simulink model "Converter_With_Parasitics_efficiency"  (R2024a)
settings: Solver=VariableStepAuto  StartTime=0.0  StopTime=0.2  RelTol=1e-3
libraries: spsSeriesRLCBranchLib x3, spsCurrentMeasurementLib x2, spsVoltageMeasurementLib x2, spsDiodeLib x1, spsMosfetLib x1, sps_lib x1, spsDCVoltageSourceLib x1
settings Model: Creator=DELL  LastModifiedBy=DELL

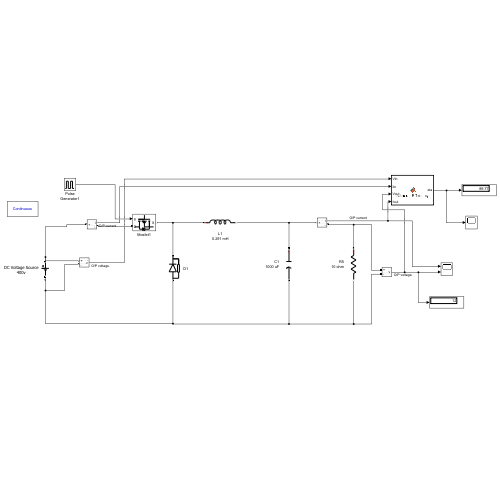
[thumbnail: Simulink's stored preview of the top-level diagram]
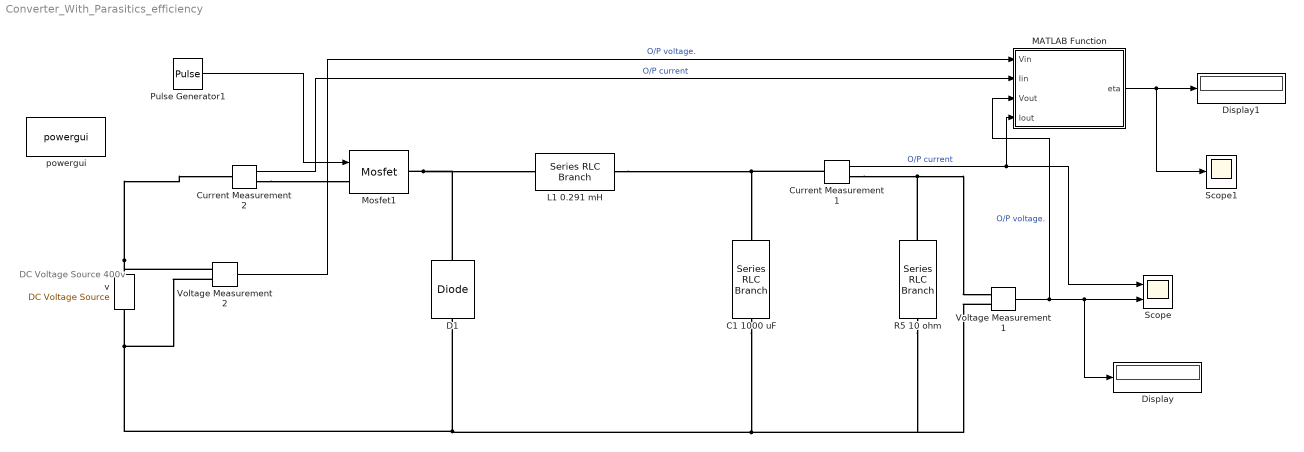
== system Converter_With_Parasitics_efficiency ==
  note: DC Voltage Source
      | 400v
  C1 1000 uF : spsSeriesRLCBranchLib/Series RLC Branch  LConnTagsString=__new0  RConnTagsString=__new0  BranchType=C  Resistance=1  Inductance=1e-3  SetiL0=off  InitialCurrent=0  Capacitance=100e-6  Setx0=off  InitialVoltage=0  Measurements=None
  Current Measurement1 : spsCurrentMeasurementLib/Current Measurement  PhasorSimulation=off  OutputType=Complex  PSBequivalent=0
  Current Measurement2 : spsCurrentMeasurementLib/Current Measurement  PhasorSimulation=off  OutputType=Complex  PSBequivalent=0
  D1 : spsDiodeLib/Diode  Ron=0.001  Lon=0  Vf=0.8  IC=0  UseSnubber=0  Rs=500  Cs=250e-9  Measurements=off
  Display : Display
  Display1 : Display
  L1 0.291 mH : spsSeriesRLCBranchLib/Series RLC Branch  LConnTagsString=__new0  RConnTagsString=__new0  BranchType=L  Resistance=1  Inductance=0.291e-3  SetiL0=off  InitialCurrent=0  Capacitance=1e-6  Setx0=off  InitialVoltage=0  Measurements=None
  MATLAB Function : MATLAB Function  TreatAsAtomicUnit=on
  Mosfet1 : spsMosfetLib/Mosfet  Ron=0.1  Lon=0  Rd=0.01  Vfd=0  IC=0  Rs=1e5  Cs=inf  Measurements=off
  Pulse Generator1 : DiscretePulseGenerator  PulseType=Time based  Period=1/200000  PulseWidth=3.1947
  R5 10 ohm : spsSeriesRLCBranchLib/Series RLC Branch  LConnTagsString=__new0  RConnTagsString=__new0  BranchType=R  Resistance=10  Inductance=1e-3  SetiL0=off  InitialCurrent=0  Capacitance=100e-6  Setx0=off  InitialVoltage=0  Measurements=None
  Scope : Scope  NumInputPorts=2
  Scope1 : Scope
  Voltage Measurement1 : spsVoltageMeasurementLib/Voltage Measurement  PhasorSimulation=off  OutputType=Complex  PSBequivalent=0
  Voltage Measurement2 : spsVoltageMeasurementLib/Voltage Measurement  PhasorSimulation=off  OutputType=Complex  PSBequivalent=0
  powergui : sps_lib/powergui  Priority=1  SimulationMode=Continuous  SampleTime=50e-6  frequency=60  Iterations=50  frequencyindice=0  Pbase=100e6  ErrMax=1e-4  UnitsV=kV  UnitsW=MW  buscounter=0  FunctionMessages=off  echomessages=off  EnableUseOfTLC=off  CurrentSourceSwitches=off  DisableSnubberDevices=off  DisableRonSwitches=off  DisableVfSwitches=off  DisplayEquations=off  AutomaticDiscreteSolvers=off  SolverType=Tustin/Backward Euler (TBE)  Interpol=off  ExternalGateDelay=off  methode=off  Ts=100  x0status=blocks  SPID=on  SwTol=0  HookPort=off  NonlinearTolerance=1e-4  nMaxIteration=100  ContinueOnMaxIteration=off  RestoreLinks=warning  ResistiveCurrentMeasurement=off  Frange=[0:2:500]  Ylog=off  Xlog=on  ShowGrid=off  save=off  variable=ZData  structure=0  ZoomFFT=off  StartTime=0.0  cycles=1  DisplayStyle=1  fundamental=60  FreqAxis=off  MaxFrequency=1000  frequencyindicesteady=1  RmsSteady=1  display=off
  v : spsDCVoltageSourceLib/DC Voltage Source  Amplitude=400  Measurements=None
  wires:
  Pulse Generator1/1 -> Mosfet1/1
  Current Measurement1/1 -> MATLAB Function/4(Iout), Scope/1  "O/P current"
  Voltage Measurement1/1 -> MATLAB Function/3(Vout), Display/1, Scope/2  "O/P voltage."
  Current Measurement2/1 -> MATLAB Function/2(Iin)  "O/P current"
  Voltage Measurement2/1 -> MATLAB Function/1(Vin)  "O/P voltage."
  MATLAB Function/1(eta) -> Scope1/1, Display1/1
  connections:
  L1 0.291 mH/RConn1 -- Current Measurement1/LConn1 -- C1 1000 uF/LConn1
  C1 1000 uF/RConn1 -- D1/LConn1 -- v/LConn1 -- Voltage Measurement2/LConn2 -- Voltage Measurement1/LConn2 -- R5 10 ohm/RConn1
  Mosfet1/RConn1 -- L1 0.291 mH/LConn1 -- D1/RConn1
  Current Measurement1/RConn1 -- Voltage Measurement1/LConn1 -- R5 10 ohm/LConn1
  v/RConn1 -- Current Measurement2/LConn1 -- Voltage Measurement2/LConn1
  Current Measurement2/RConn1 -- Mosfet1/LConn1

== matlab function Converter_With_Parasitics_efficiency/MATLAB Function ==
  data: Vin input; eta output; Iin input; Vout input; Iout input
function eta = calculateEfficiency(Vin, Iin, Vout, Iout)

    % Ensure all inputs are column vectors
    Vin = Vin(:);
    Iin = Iin(:);
    Vout = Vout(:);
    Iout = Iout(:);

    % Instantaneous powers
    Pin = Vin .* Iin;
    Pout = Vout .* Iout;

    % Handle sign issues
    Pin_avg = abs(mean(Pin));
    Pout_avg = mean(Pout);

    % Prevent divide-by-zero
    if Pin_avg < 1e-3
        warning('Input power is too low. Check input current.');
        eta = 0;
    else
        eta = (Pout_avg / Pin_avg) *10;
    end

    fprintf('Efficiency: %.2f %%\n', eta);
end
